simulink model "sim_tan"  (R2018a)
settings: Solver=ode45  StartTime=0.0  StopTime=3000  RelTol=1e-3
InitFcn:
  | codigo_ex
values from neighbouring files (symbols this model uses):
  Ad = [0.9888    0.0001    0.0112 ... (first row only)    [proceso.m]
  Bd = [64.5687    0.0014 ... (first row only)    [proceso.m]
  Cd = eye(3)    [codigo_ex.m]    (also in sistema_tanques_control.m; tank_mod.m)
  K1 = [21.6 3 -5; 2.9 19 -4]*10e-4    [codigo_ex.m]    (also in controlador.m = [0.0216    0.0030   -0.0050; prueba_controlador_cpp.m = [0.0216    0.0030   -0.0050; sistema_tanques_control.m; tank_mod.m)
  K2 = [-0.95 -0.32; -0.3 -0.91]*10e-4    [codigo_ex.m]    (also in controlador.m = 1.0e-03 *K2; prueba_controlador_cpp.m = 1.0e-03 *K2; sistema_tanques_control.m; tank_mod.m)
  q_max = 1.5*10e-4    (= 0.0015)    [codigo_ex.m]    (also in controlador.m; prueba_controlador_cpp.m; sistema_tanques_control.m; tank_mod.m)
  q_min = 0    [codigo_ex.m]    (also in controlador.m; prueba_controlador_cpp.m; sistema_tanques_control.m; tank_mod.m)
  tm = 1    [codigo_ex.m]    (also in sistema_tanques_control.m; tank_mod.m)
settings Model: Creator=cmparedes  LastModifiedBy=carma

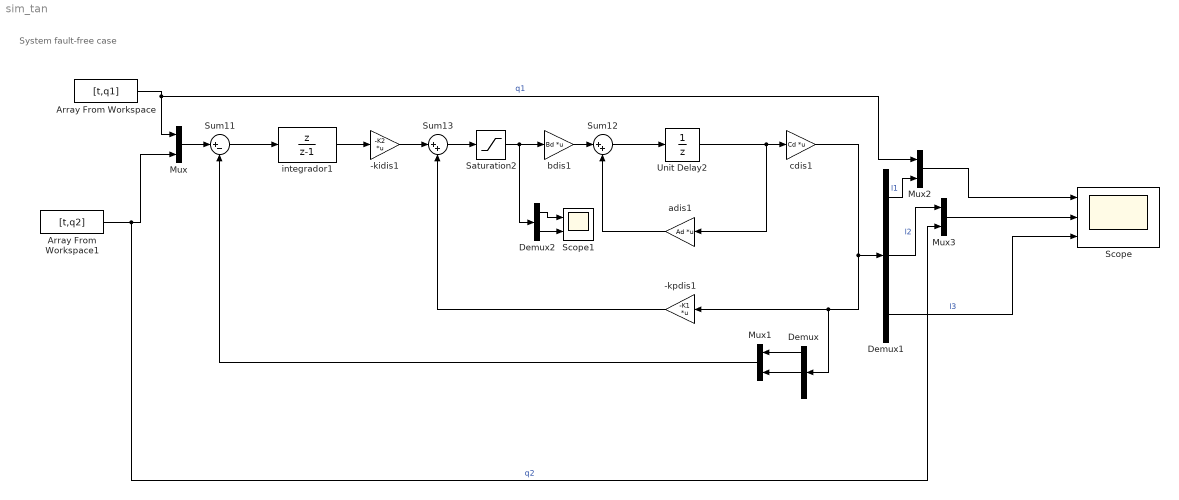
== system sim_tan ==
  note: System fault-free case
  -kidis1 : Gain  Gain=-K2  Multiplication=Matrix(K*u) (u vector)  SampleTime=tm
  -kpdis1 : Gain  Gain=-K1  Multiplication=Matrix(K*u) (u vector)  SampleTime=tm
  Array From Workspace : FromWorkspace  VariableName=[t,q1]  SampleTime=0
  Array From Workspace1 : FromWorkspace  VariableName=[t,q2]  SampleTime=0
  Demux : Demux  Outputs=3
  Demux1 : Demux  Outputs=3
  Demux2 : Demux  Outputs=2
  Mux{,1..3} (4 alike) : Mux  Inputs=2
  Saturation2 : Saturate  UpperLimit=q_max  LowerLimit=q_min
  Scope : Scope  NumInputPorts=3
  Scope1 : Scope  NumInputPorts=2
  Sum11 : Sum  Inputs=|+-  SampleTime=tm
  Sum12 : Sum  Inputs=|++  SampleTime=tm
  Sum13 : Sum  Inputs=|++  SampleTime=tm
  Unit Delay2 : UnitDelay  SampleTime=tm
  adis1 : Gain  Gain=Ad  Multiplication=Matrix(K*u) (u vector)  SampleTime=tm
  bdis1 : Gain  Gain=Bd  Multiplication=Matrix(K*u) (u vector)  SampleTime=tm
  cdis1 : Gain  Gain=Cd  Multiplication=Matrix(K*u) (u vector)  SampleTime=tm
  integrador1 : DiscreteTransferFcn  Numerator=[1 0]  Denominator=[1 -1]  SampleTime=tm
  wires:
  -kidis1/1 -> Sum13/1
  adis1/1 -> Sum12/2
  Sum12/1 -> Unit Delay2/1
  Sum11/1 -> integrador1/1
  integrador1/1 -> -kidis1/1
  -kpdis1/1 -> Sum13/2
  bdis1/1 -> Sum12/1
  Mux/1 -> Sum11/1
  Demux/1 -> Mux1/1
  Mux1/1 -> Sum11/2
  cdis1/1 -> Demux1/1, -kpdis1/1, Demux/1
  Demux/2 -> Mux1/2
  Demux2/1 -> Scope1/1
  Demux2/2 -> Scope1/2
  Demux1/1 -> Mux2/2  "l1"
  Mux2/1 -> Scope/1
  Demux1/2 -> Mux3/1  "l2"
  Mux3/1 -> Scope/2
  Demux1/3 -> Scope/3  "l3"
  Array From Workspace/1 -> Mux2/1, Mux/1  "q1"
  Array From Workspace1/1 -> Mux3/2, Mux/2  "q2"
  Sum13/1 -> Saturation2/1
  Unit Delay2/1 -> adis1/1, cdis1/1
  Saturation2/1 -> Demux2/1, bdis1/1
